simulink subsystem "heat_sink"  (R2020b)
settings: Solver=VariableStepAuto  StartTime=0.0  StopTime=10.0  RelTol=1e-3
model mask{fidelityPARAM=Reduced Order Model, romPARAM=ROM.mat}
  mask prompts: fidelityPARAM "Choose fidelity:"; romPARAM "ROM file:"
undefined symbols (not defined in the file): h_forced, h_free, IC, normalizedForcedBC, normalizedFreeBC, rsys, sys, Tinf, unitCPUHeat, unitForcedBC, unitFreeBC
settings Model: Creator=jclinton  LastModifiedBy=jclinton
settings DebuggingCC: SFMachineParentedDataDiag=error

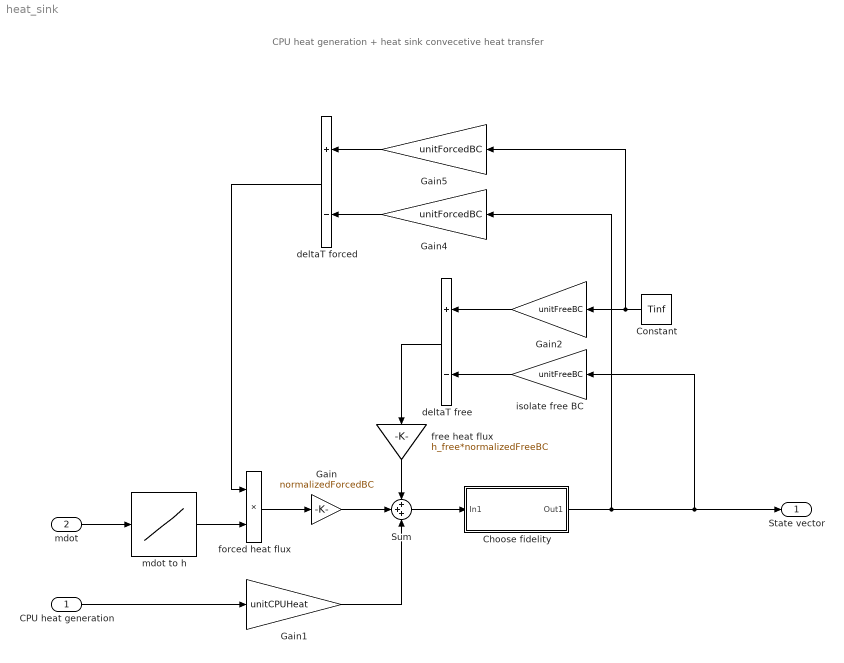
== system heat_sink ==
  note: CPU heat generation + heat sink convecetive heat transfer
  CPU heat generation : Inport  Unit=W
  mdot : Inport  Port=2  Unit=kg/sec
  Choose fidelity : Subsystem  Variant=on  VariantControlMode=label  LabelModeActiveChoice=Choice_2
      mask init:
      | fidelity = get_param(gcs,'fidelityPARAM');
      | vssBlk = gcb;
      | if strcmp(fidelity,'Finite Element Model')
      |     set_param(vssBlk, 'LabelModeActiveChoice', 'Choice_1');
      | else
      |     set_param(vssBlk, 'LabelModeActiveChoice', 'Choice_2');
      |     romfile = get_param(gcs,'romPARAM');
      |     topdir = evalin('base','topdir');
      |     load([topdir filesep 'data' filesep romfile],'rsys');
      |     assignin('base','rsys',rsys);
      | end
      mask DialogControl DescGroupVar Prompt: Choose between FE formulation or a reduced order model
      mask DialogControl DescTextVar Prompt: Different DSS blocks underneath mask chosen depending on desirede fidelity
      mask Display: disp('\partialu/\partialt = \alpha(\Deltau)','texmode','on')
  Constant : Constant  Value=Tinf
  Gain : Gain  Gain=normalizedForcedBC
  Gain1 : Gain  Gain=unitCPUHeat
  Gain2 : Gain  Gain=unitFreeBC
  Gain4 : Gain  Gain=unitForcedBC
  Gain5 : Gain  Gain=unitForcedBC
  Sum : Sum  Inputs=+++
  "deltaT forced " : Sum  Inputs=+-
  deltaT free : Sum  Inputs=+-
  forced heat flux : Product
  free heat flux : Gain  Gain=h_free*normalizedFreeBC
  isolate free BC : Gain  Gain=unitFreeBC
  mdot to h : Lookup_n-D  NumberOfTableDimensions=1  BreakpointsForDimension1=h_forced(:,1)  Table=h_forced(:,2)  InternalRulePriority=Speed  RndMeth=Simplest  InputSameDT=on
  State vector : Outport  Unit=K
  wires:
  mdot/1 -> mdot to h/1
  mdot to h/1 -> forced heat flux/2
  forced heat flux/1 -> Gain/1
  Gain/1 -> Sum/2
  free heat flux/1 -> Sum/1
  deltaT free/1 -> free heat flux/1
  Gain2/1 -> deltaT free/1
  Constant/1 -> Gain5/1, Gain2/1
  isolate free BC/1 -> deltaT free/2
  Gain4/1 -> "deltaT forced "/2
  Gain5/1 -> "deltaT forced "/1
  "deltaT forced "/1 -> forced heat flux/1
  CPU heat generation/1 -> Gain1/1
  Gain1/1 -> Sum/3
  Choose fidelity/1(Out1) -> Gain4/1, State vector/1, isolate free BC/1
  Sum/1 -> Choose fidelity/1(In1)

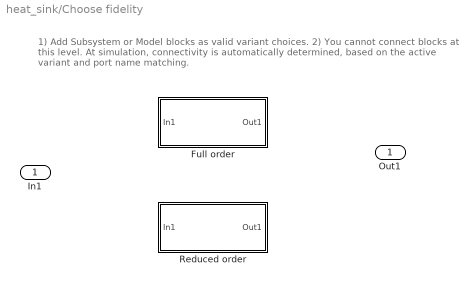
== system heat_sink/Choose fidelity ==
  note: 1) Add Subsystem or Model blocks as valid variant choices.
      | 2) You cannot connect blocks at this level. At simulation, connectivity is automatically
      | determined, based on the active variant and port name matching.
  In1 : Inport
  Full order : Subsystem  VariantControl=Choice_1
  Reduced order : Subsystem  VariantControl=Choice_2
  Out1 : Outport

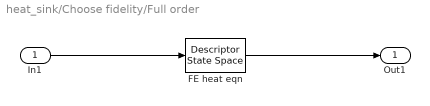
== system heat_sink/Choose fidelity/Full order ==
  In1 : Inport
  FE heat eqn : DescriptorStateSpace  E=sys.E  A=-sys.A  B=sys.B  C=sys.C  D=sys.D  InitialCondition=IC  DirectFeedthrough=False
  Out1 : Outport
  wires:
  FE heat eqn/1 -> Out1/1
  In1/1 -> FE heat eqn/1

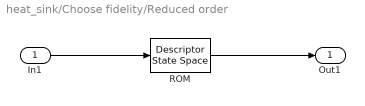
== system heat_sink/Choose fidelity/Reduced order ==
  In1 : Inport
  ROM : DescriptorStateSpace  E=rsys.E  A=-rsys.A  B=rsys.B  C=rsys.C  D=rsys.D  InitialCondition=IC  DirectFeedthrough=False
  Out1 : Outport
  wires:
  ROM/1 -> Out1/1
  In1/1 -> ROM/1
